simulink model "esp_siml"  (R2020b)
settings: Solver=VariableStepAuto  StartTime=0.0  StopTime=7.1  RelTol=1e-3
values from neighbouring files (symbols this model uses):
  A = [1.0000    0.1000;0    1.0000]    [RLenv.m]    (also in RlEnvModel.m; envRL.mat = [1  0.1; 0  1]; sys_env.m)
  B = [0.0050;0.1000]    [RLenv.m]    (also in RlEnvModel.m; envRL.mat = [0.005 0.1]; sys_env.m)
  C = [1 0]    [RLenv.m]    (also in RlEnvModel.m; envRL.mat; sys_env.m)
  D = [0]    [RLenv.m]    (also in RlEnvModel.m; envRL.mat = 0; sys_env.m)
  K = [16.0302    5.6622]    [RLenv.m]    (also in RlEnvModel.m; envRL.mat = [16.0302 5.6622]; sys_env.m)
  L = [0.9902;0.9892]    [RLenv.m]    (also in RlEnvModel.m; envRL.mat = [0.9902 0.9892]; sys_env.m)
  Ts = 0.1    [RLenv.m]    (also in RlEnvModel.m; envRL.mat; sys_env.m)
libraries: simulink x2
settings Model: Creator=Shreyash  LastModifiedBy=IIT_KGP_CSE_FM_LAB
settings DataIOCC: ReturnWorkspaceOutputs=off
settings DebuggingCC: ArithmeticOperatorsInVariantConditions=warning
settings SFSimCC: SimUseLocalCustomCode=off  CustomCodeUndefinedFunction=UseInterfaceOnly
settings RTWCC: RTWUseLocalCustomCode=off

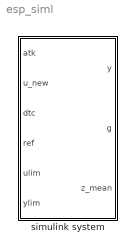
== system esp_siml ==
  simulink system : Subsystem

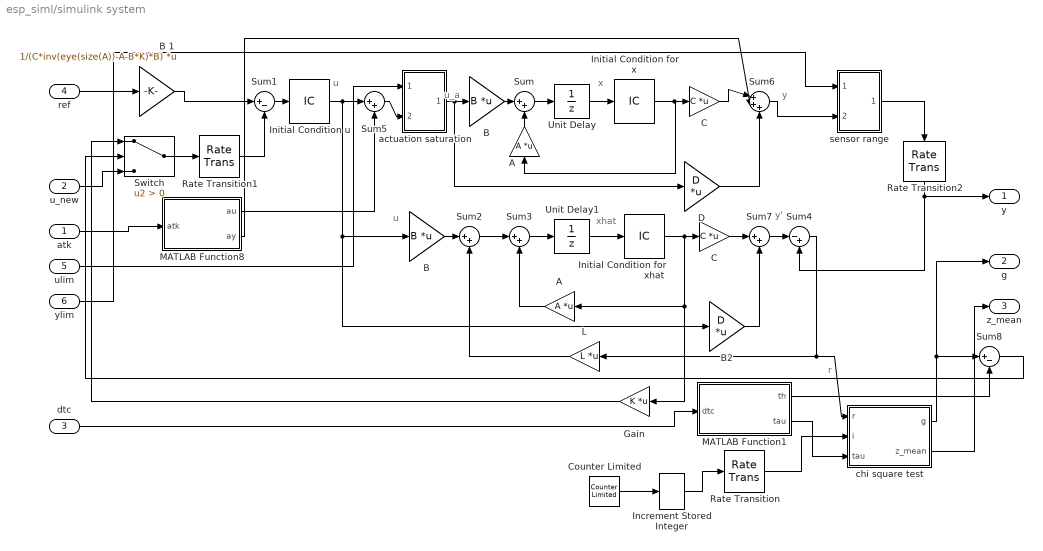
== system esp_siml/simulink system ==
  note: y
  note: r
  note: y'
  note: u
  note: u
  note: x
  note: xhat
  note: u_a
  atk : Inport
  u_new : Inport  Port=2
  dtc : Inport  Port=3
  ref : Inport  Port=4
  ulim : Inport  Port=5
  ylim : Inport  Port=6
  A : Gain  Gain=A  Multiplication=Matrix(K*u)
  "A " : Gain  Gain=A  Multiplication=Matrix(K*u)
  B : Gain  Gain=B  Multiplication=Matrix(K*u)
  "B " : Gain  Gain=B  Multiplication=Matrix(K*u)
  B 1 : Gain  Gain=1/(C*inv(eye(size(A))-A-B*K)*B)  Multiplication=Matrix(K*u)
  B2 : Gain  Gain=D  Multiplication=Matrix(K*u)
  C : Gain  Gain=C  Multiplication=Matrix(K*u)
  "C " : Gain  Gain=C  Multiplication=Matrix(K*u)
  Counter Limited : simulink/Sources/Counter Limited  uplimit=1/Ts-1  tsamp=Ts
  D : Gain  Gain=D  Multiplication=Matrix(K*u)
  Gain : Gain  Gain=K  Multiplication=Matrix(K*u)
  Increment Stored Integer : simulink/Additional Math & Discrete/Additional Math: Increment - Decrement/Increment Stored Integer
  Initial Condition u : InitialCondition  Value=zeros(size(B,2),1)
  Initial Condition for x : InitialCondition  Value=[0;0]
  Initial Condition for xhat : InitialCondition  Value=[0;0]
  L : Gain  Gain=L  Multiplication=Matrix(K*u)
  MATLAB Function1 : MATLAB Function  TreatAsAtomicUnit=on
  MATLAB Function8 : MATLAB Function  TreatAsAtomicUnit=on
  Rate Transition : RateTransition  OutPortSampleTime=Ts
  Rate Transition1 : RateTransition  OutPortSampleTime=Ts
  Rate Transition2 : RateTransition  OutPortSampleTime=Ts
  Sum{,2..3,5,7} (5 alike) : Sum  Inputs=|++
  Sum1 : Sum  Inputs=|+-
  Sum4 : Sum  Inputs=|-+
  Sum6 : Sum  Inputs=|+++
  Sum8 : Sum  Inputs=|+-
  Switch : Switch  Criteria=u2 > Threshold
  Unit Delay : UnitDelay  SampleTime=-1  HasFrameUpgradeWarning=on
  Unit Delay1 : UnitDelay  SampleTime=-1  HasFrameUpgradeWarning=on
  actuation saturation : Subsystem
  chi square test : Subsystem
  sensor range : Subsystem
  y : Outport
  g : Outport  Port=2
  z_mean : Outport  Port=3
  wires:
  Initial Condition for xhat/1 -> C/1, A/1, Gain/1
  L/1 -> Sum2/2
  "C "/1 -> Sum6/1
  D/1 -> Sum6/3
  u_new/1 -> Switch/3
  Unit Delay1/1 -> Initial Condition for xhat/1
  Sum7/1 -> Sum4/1
  Sum4/1 -> chi square test/1(r), L/1
  Sum3/1 -> Unit Delay1/1
  Unit Delay/1 -> Initial Condition for x/1
  Sum2/1 -> Sum3/1
  Sum1/1 -> Initial Condition u/1
  Initial Condition u/1 -> B/1, B2/1, Sum5/1
  Gain/1 -> Switch/1
  B2/1 -> Sum7/2
  actuation saturation/1(Out1) -> D/1, "B "/1
  A/1 -> Sum3/2
  Sum5/1 -> actuation saturation/2(In3)
  "B "/1 -> Sum/1
  Sum6/1 -> sensor range/2(In3)
  C/1 -> Sum7/1
  "A "/1 -> Sum/2
  Initial Condition for x/1 -> "C "/1, "A "/1
  ref/1 -> B 1/1
  B/1 -> Sum2/1
  Switch/1 -> Rate Transition1/1
  Sum/1 -> Unit Delay/1
  Sum8/1 -> Switch/2
  atk/1 -> MATLAB Function8/1(atk)
  MATLAB Function8/1(au) -> Sum5/2
  MATLAB Function8/2(ay) -> Sum6/2
  B 1/1 -> Sum1/1
  dtc/1 -> MATLAB Function1/1(dtc)
  MATLAB Function1/2(tau) -> chi square test/3(tau)
  chi square test/1(g) -> g/1, Sum8/1
  MATLAB Function1/1(th) -> Sum8/2
  ulim/1 -> actuation saturation/1(lim)
  sensor range/1(y_obs) -> Rate Transition2/1
  ylim/1 -> sensor range/1(lim)
  chi square test/2(z_mean) -> z_mean/1
  Increment Stored Integer/1 -> Rate Transition/1
  Counter Limited/1 -> Increment Stored Integer/1
  Rate Transition/1 -> chi square test/2(i)
  Rate Transition1/1 -> Sum1/2
  Rate Transition2/1 -> y/1, Sum4/2

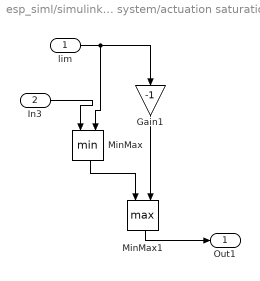
== system esp_siml/simulink system/actuation saturation ==
  lim : Inport
  In3 : Inport  Port=2
  Gain1 : Gain  Gain=-1
  MinMax : MinMax  Inputs=2
  MinMax1 : MinMax  Function=max  Inputs=2
  Out1 : Outport
  wires:
  Gain1/1 -> MinMax1/2
  MinMax/1 -> MinMax1/1
  MinMax1/1 -> Out1/1
  lim/1 -> Gain1/1, MinMax/2
  In3/1 -> MinMax/1

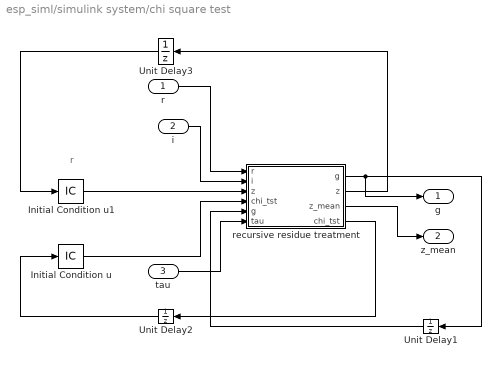
== system esp_siml/simulink system/chi square test ==
  note: r
  r : Inport
  i : Inport  Port=2
  tau : Inport  Port=3
  Initial Condition u : InitialCondition  Value=[0]
  Initial Condition u1 : InitialCondition  Value=[0]
  Unit Delay1 : UnitDelay  SampleTime=Ts  HasFrameUpgradeWarning=on
  Unit Delay2 : UnitDelay  SampleTime=Ts  HasFrameUpgradeWarning=on
  Unit Delay3 : UnitDelay  InitialCondition=[0]  SampleTime=Ts  HasFrameUpgradeWarning=on
  recursive residue treatment : MATLAB Function  TreatAsAtomicUnit=on
  g : Outport
  z_mean : Outport  Port=2
  wires:
  Unit Delay2/1 -> Initial Condition u/1
  Initial Condition u1/1 -> recursive residue treatment/3("z ")
  r/1 -> recursive residue treatment/1(r)
  Unit Delay1/1 -> recursive residue treatment/5("g ")
  Initial Condition u/1 -> recursive residue treatment/4("chi_tst ")
  Unit Delay3/1 -> Initial Condition u1/1
  recursive residue treatment/3(z_mean) -> z_mean/1
  i/1 -> recursive residue treatment/2(i)
  recursive residue treatment/4(chi_tst) -> Unit Delay2/1
  tau/1 -> recursive residue treatment/6(tau)
  recursive residue treatment/2(z) -> Unit Delay3/1
  recursive residue treatment/1(g) -> Unit Delay1/1, g/1

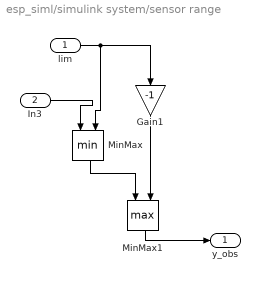
== system esp_siml/simulink system/sensor range ==
  lim : Inport
  In3 : Inport  Port=2
  Gain1 : Gain  Gain=-1
  MinMax : MinMax  Inputs=2
  MinMax1 : MinMax  Function=max  Inputs=2
  y_obs : Outport
  wires:
  Gain1/1 -> MinMax1/2
  MinMax/1 -> MinMax1/1
  MinMax1/1 -> y_obs/1
  lim/1 -> Gain1/1, MinMax/2
  In3/1 -> MinMax/1

== matlab function esp_siml/simulink system/MATLAB Function1 ==
  data: th output; dtc input; tau output
function [th,tau] = dtcParams(dtc)
    th= dtc(1);
    tau= dtc(2);

== matlab function esp_siml/simulink system/MATLAB Function8 ==
  data: au output; atk input; ay output
function [au,ay] = atkParams(atk)
    au= atk(1);
    ay= atk(2);

== matlab function esp_siml/simulink system/chi square test/recursive residue treatment ==
  data: g output; r input; i input; z input; z output; z_mean output; chi_tst output; chi_tst input; g input; tau input
function [g,z,z_mean,chi_tst] = fcn(r,i,z,chi_tst,g,tau)
i
z(i)=r
z_mean=mean(z)
P= size(z',1)
chi_tst(i)= z(:,i)'*z(:,i)/P
g(i) = 0;              
for k = max(1,i-tau+1):i
    g(i) = g(i) + chi_tst(k)  % Calculate gk (chi2 test)
end
